simulink model "original_controller"  (R2016a)
settings: Solver=VariableStepAuto  StartTime=0.0  StopTime=5000  RelTol=1e-3
values from neighbouring files (symbols this model uses):
  A = [0 .01 ; 0 -.001]    [PnPC.m]
  B = [6.25 0 -1 ; 0 10 0]    [PnPC.m]
  C = [1 0]    [PnPC.m]
libraries: simulink x1, cstblocks x1
settings Model: Creator=Linda und Andreas  LastModifiedBy=Linda und Andreas

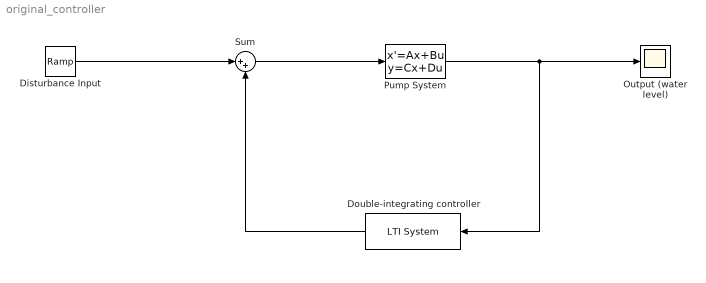
== system original_controller ==
  Disturbance Input : simulink/Sources/Ramp  slope=[0;0;1]  start=5  X0=[0;0;0]  VectorParams1D=off
  Double-integrating controller : cstblocks/LTI System  sys=K0  IC=[]
  Output (water level) : Scope
  Pump System : StateSpace  A=A  B=B  C=C  D=[0 0 0]  X0=0
  Sum : Sum  Inputs=|++
  wires:
  Double-integrating controller/1 -> Sum/2
  Sum/1 -> Pump System/1
  Pump System/1 -> Double-integrating controller/1, Output (water level)/1
  Disturbance Input/1 -> Sum/1
